simulink model "Junctions6"  (Simulink 5.0)
settings: Solver=ode45  StartTime=0.0  StopTime=10.0  RelTol=1e-3
settings Model: Creator=scaife  LastModifiedBy=scaife  ExtModeAutoUpdateStatusClock=off

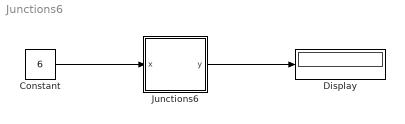
== system Junctions6 ==
  Constant : Constant  Value=6
  Display : Display
  Junctions6 : Stateflow chart
  wires:
  Constant/1 -> Junctions6/1(x)
  Junctions6/1(y) -> Display/1

== stateflow chart Junctions6 ==
  state TOP
    state A
    state B
    state C
    state D
    (default) -> A : [x<4]{y+=1}
    (default) -> B : [x>=4]{y+=10}
    A -> (junction 8) : [x<=2]{y+=100}
    B -> (junction 8) : [x>=6]{y+=1000}
    (junction 8) -> C : [x %% 3 == 1]{y+=10000}
    (junction 8) -> D : [x %% 3 == 0]{y+=100000}
    D -> C : [1]
    C -> TOP
  (default) -> TOP
  data: x input int32; y output int32 =111111
